simulink model "HighPassFilter"  (R2020b)
settings: Solver=FixedStepAuto  StartTime=0.0  StopTime=50  FixedStep=0.0001  RelTol=1e-3
settings Model: Creator=baner  LastModifiedBy=baner

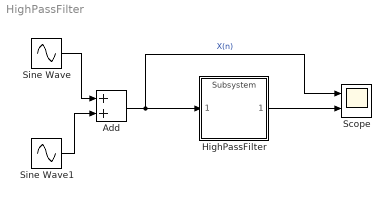
== system HighPassFilter ==
  Add : Sum
  HighPassFilter : ModelReference  ModelNameDialog=Subsystem  SimulationMode=Normal  ModelReferenceVersion=1.3
  Scope : Scope  NumInputPorts=2
  Sine Wave : Sin  Frequency=1000  SampleTime=0
  Sine Wave1 : Sin  Amplitude=2  Frequency=4  SampleTime=0
  wires:
  Add/1 -> Scope/1, HighPassFilter/1  "X(n)"
  HighPassFilter/1 -> Scope/2
  Sine Wave/1 -> Add/1
  Sine Wave1/1 -> Add/2
